simulink model "ADPLL_c7"  (R2017a)
settings: Solver=VariableStepAuto  StartTime=0.0  StopTime=4e-4  FixedStep=1/(12*4*Fref)  RelTol=1e-3
values from neighbouring files (symbols this model uses):
  BBPFD_delay = 1e-09    [processed_29-Aug-2018 09_50_30.mat]    (also in search_0_Kdco-0.9e6_Nref-1e-19_Ndco-1e12.mat; search_0_Kdco-1.0e6_Nref-1e-19_Ndco-1e11.mat; search_0_Kdco-1.0e6_Nref-1e-19_Ndco-1e12.mat; search_0_Kdco-1.0e6_Nref-1e-19_Ndco-1e13.mat)
  DCO_Noise = Datas(i,3)    [CreateDatasetv3.m]    (also in CreateDatasetv4.m; search_0_Kdco-0.9e6_Nref-1e-19_Ndco-1e12.mat = 1000000000000; search_0_Kdco-1.0e6_Nref-1e-19_Ndco-1e11.mat = 100000000000; search_0_Kdco-1.0e6_Nref-1e-19_Ndco-1e12.mat = 1000000000000)
  DCO_Seed = DCO_Seed+1    [CreateDatasetv2.m]    (also in CreateDatasetv3.m = 1; CreateDatasetv4.m = 1; processed_29-Aug-2018 09_50_30.mat = 1; search_0_Kdco-0.9e6_Nref-1e-19_Ndco-1e12.mat = 65)
  Ffree = 255000000    [processed_29-Aug-2018 09_50_30.mat]    (also in search_0_Kdco-0.9e6_Nref-1e-19_Ndco-1e12.mat = 250000000; search_0_Kdco-1.0e6_Nref-1e-19_Ndco-1e11.mat = 250000000; search_0_Kdco-1.0e6_Nref-1e-19_Ndco-1e12.mat = 250000000; search_0_Kdco-1.0e6_Nref-1e-19_Ndco-1e13.mat = 250000000)
  Fref = 25500000    [processed_29-Aug-2018 09_50_30.mat]    (also in search_0_Kdco-0.9e6_Nref-1e-19_Ndco-1e12.mat = 25000000; search_0_Kdco-1.0e6_Nref-1e-19_Ndco-1e11.mat = 25000000; search_0_Kdco-1.0e6_Nref-1e-19_Ndco-1e12.mat = 25000000; search_0_Kdco-1.0e6_Nref-1e-19_Ndco-1e13.mat = 25000000)
  K3 = Datas(i,4)    [CreateDatasetv3.m]    (also in CreateDatasetv4.m)
  K4 = Datas(i,5)    [CreateDatasetv3.m]    (also in CreateDatasetv4.m)
  Kdco = Datas(i,1)    [CreateDatasetv3.m]    (also in CreateDatasetv4.m; search_0_Kdco-0.9e6_Nref-1e-19_Ndco-1e12.mat = 900000; search_0_Kdco-1.0e6_Nref-1e-19_Ndco-1e11.mat = 1000000; search_0_Kdco-1.0e6_Nref-1e-19_Ndco-1e12.mat = 1000000)
  Ki = 0.01    [processed_29-Aug-2018 09_50_30.mat]    (also in search_0_Kdco-0.9e6_Nref-1e-19_Ndco-1e12.mat; search_0_Kdco-1.0e6_Nref-1e-19_Ndco-1e11.mat; search_0_Kdco-1.0e6_Nref-1e-19_Ndco-1e12.mat; search_0_Kdco-1.0e6_Nref-1e-19_Ndco-1e13.mat)
  N = 10    [processed_29-Aug-2018 09_50_30.mat]    (also in search_0_Kdco-0.9e6_Nref-1e-19_Ndco-1e12.mat; search_0_Kdco-1.0e6_Nref-1e-19_Ndco-1e11.mat; search_0_Kdco-1.0e6_Nref-1e-19_Ndco-1e12.mat; search_0_Kdco-1.0e6_Nref-1e-19_Ndco-1e13.mat)
  Ref_Noise = Datas(i,2)    [CreateDatasetv3.m]    (also in CreateDatasetv4.m; search_0_Kdco-0.9e6_Nref-1e-19_Ndco-1e12.mat = 1e-19; search_0_Kdco-1.0e6_Nref-1e-19_Ndco-1e11.mat = 1e-19; search_0_Kdco-1.0e6_Nref-1e-19_Ndco-1e12.mat = 1e-19)
  Ref_Seed = Ref_Seed+1    [CreateDatasetv2.m]    (also in CreateDatasetv3.m = 0; CreateDatasetv4.m = 0; processed_29-Aug-2018 09_50_30.mat = 0; search_0_Kdco-0.9e6_Nref-1e-19_Ndco-1e12.mat = 64)
undefined symbols (not defined in the file): Kp
libraries: simulink_extras x3, dspswit3 x2, simulink x2
settings Model: Creator=ECL328  LastModifiedBy=ECL328

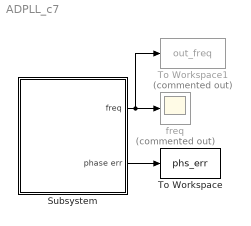
== system ADPLL_c7 ==
  Subsystem : Subsystem  mask{N=N, Kp=Kp, Ki=Ki, Kdco=Kdco, Fref=Fref, Ffree=Ffree, BBPFD_delay=BBPFD_delay, Ref_Noise=Ref_Noise, DCO_Noise=DCO_Noise}
      mask prompts: Ref_Noise "Var of RefNoise"; DCO_Noise "Var of DCONoise"
  To Workspace : ToWorkspace  VariableName=phs_err  SampleTime=-1
  To Workspace1 : ToWorkspace  Commented=on  VariableName=out_freq  SampleTime=-1
  freq : Scope  Commented=on
  wires:
  Subsystem/1(freq) -> To Workspace1/1, freq/1
  Subsystem/2(phase err) -> To Workspace/1

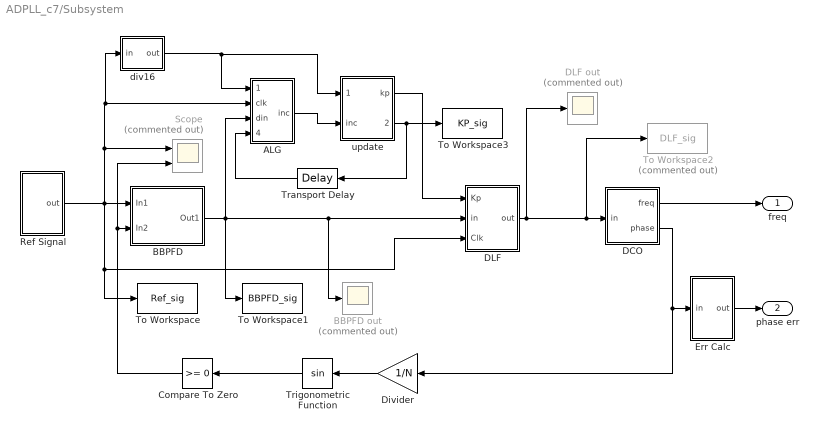
== system ADPLL_c7/Subsystem ==
  ALG : Subsystem
  BBPFD : Subsystem
  BBPFD out : Scope  Commented=on
  Compare To Zero : simulink/Logic and Bit Operations/Compare To Zero  relop=>=  OutDataTypeStr=boolean
  DCO : Subsystem
  DLF : Subsystem
  DLF out : Scope  Commented=on
  Divider : Gain  Gain=1/N
  Err Calc : Subsystem
  Ref Signal : Subsystem
  Scope : Scope  Commented=on  NumInputPorts=2
  To Workspace : ToWorkspace  VariableName=Ref_sig  SampleTime=-1
  To Workspace1 : ToWorkspace  VariableName=BBPFD_sig  SampleTime=-1
  To Workspace2 : ToWorkspace  Commented=on  VariableName=DLF_sig  SampleTime=-1
  To Workspace3 : ToWorkspace  VariableName=KP_sig  SampleTime=-1
  Transport Delay : TransportDelay  DelayTime=BBPFD_delay
  Trigonometric Function : Trigonometry
  div16 : Subsystem
  update : Subsystem
  freq : Outport
  phase err : Outport  Port=2
  wires:
  BBPFD/1(Out1) -> ALG/3(din), To Workspace1/1, DLF/2(in), BBPFD out/1
  Divider/1 -> Trigonometric Function/1
  DLF/1(out) -> DLF out/1, To Workspace2/1, DCO/1(in)
  DCO/1(freq) -> freq/1
  Ref Signal/1(out) -> To Workspace/1, DLF/3(Clk), div16/1(in), ALG/2(clk), Scope/1, BBPFD/1(In1)
  Err Calc/1(out) -> phase err/1
  DCO/2(phase) -> Err Calc/1(in), Divider/1
  Trigonometric Function/1 -> Compare To Zero/1
  Compare To Zero/1 -> Scope/2, BBPFD/2(In2)
  update/1(kp) -> DLF/1(Kp)
  ALG/1(inc) -> update/2(inc)
  update/2(kpraw) -> Transport Delay/1, To Workspace3/1
  Transport Delay/1 -> ALG/4(kpraw)
  div16/1(out) -> update/1("clk16 "), ALG/1(clk16)

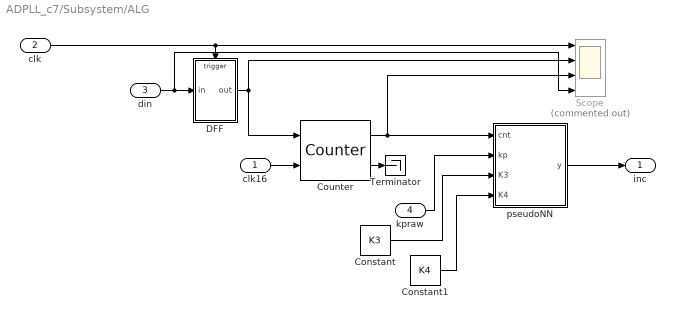
== system ADPLL_c7/Subsystem/ALG ==
  clk16 : Inport
  clk : Inport  Port=2
  din : Inport  Port=3
  kpraw : Inport  Port=4
  Constant : Constant  Value=K3
  Constant1 : Constant  Value=K4
  Counter : dspswit3/Counter  Direction=Up  CountEvent=Rising edge  CounterSize=User defined  MaxCount=1024  InitialCount=0  Output=Count and Hit  HitValue=1024  ResetInput=on  SamplesPerFrame=1  Ts=1  CntDtype=double  HitDtype=Logical
  DFF : Subsystem
  Scope : Scope  Commented=on  NumInputPorts=4
  Terminator : Terminator
  pseudoNN : MATLAB Function  TreatAsAtomicUnit=on
  inc : Outport
  wires:
  Counter/2 -> Terminator/1
  din/1 -> Scope/4, DFF/1(in)
  clk/1 -> Scope/1, DFF/Trigger
  DFF/1(out) -> Scope/2, Counter/1
  Counter/1 -> pseudoNN/1(cnt), Scope/3
  pseudoNN/1(y) -> inc/1
  kpraw/1 -> pseudoNN/2(kp)
  clk16/1 -> Counter/2
  Constant/1 -> pseudoNN/3(K3)
  Constant1/1 -> pseudoNN/4(K4)

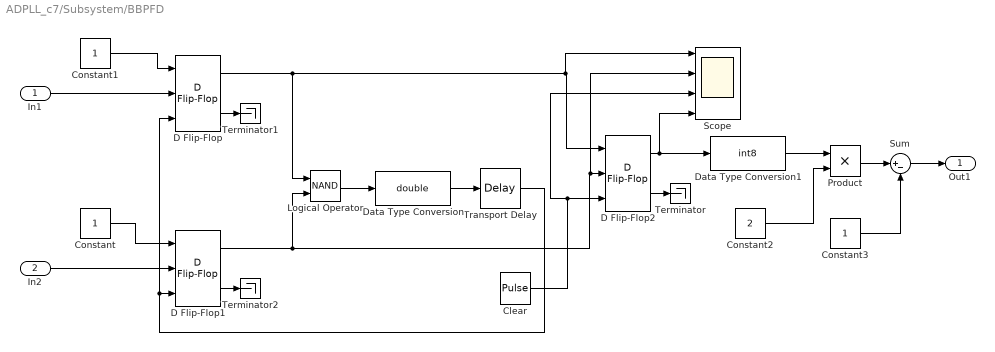
== system ADPLL_c7/Subsystem/BBPFD ==
  In1 : Inport
  In2 : Inport  Port=2
  Clear : DiscretePulseGenerator  PulseType=Time based  Period=20  PulseWidth=50
  Constant : Constant  OutDataTypeStr=boolean
  Constant1 : Constant  OutDataTypeStr=boolean
  Constant2 : Constant  Value=2
  Constant3 : Constant
  D Flip-Flop : simulink_extras/Flip Flops/D Flip-Flop
      settings: SourceProductName=Simulink
  D Flip-Flop1 : simulink_extras/Flip Flops/D Flip-Flop
      settings: SourceProductName=Simulink
  D Flip-Flop2 : simulink_extras/Flip Flops/D Flip-Flop
      settings: SourceProductName=Simulink
  Data Type Conversion : DataTypeConversion  OutDataTypeStr=double
  Data Type Conversion1 : DataTypeConversion  OutDataTypeStr=int8
  Logical Operator : Logic  Operator=NAND  AllPortsSameDT=off  OutDataTypeStr=boolean
  Product : Product
  Scope : Scope  NumInputPorts=4
  Sum : Sum  Inputs=|+-
  Terminator : Terminator
  Terminator1 : Terminator
  Terminator2 : Terminator
  Transport Delay : TransportDelay  DelayTime=BBPFD_delay
  Out1 : Outport
  wires:
  Data Type Conversion/1 -> Transport Delay/1
  Constant/1 -> D Flip-Flop1/1
  Sum/1 -> Out1/1
  D Flip-Flop2/1 -> Scope/4, Data Type Conversion1/1
  Product/1 -> Sum/1
  In1/1 -> D Flip-Flop/2
  Clear/1 -> Scope/3, D Flip-Flop2/3
  D Flip-Flop2/2 -> Terminator/1
  In2/1 -> D Flip-Flop1/2
  Constant3/1 -> Sum/2
  Data Type Conversion1/1 -> Product/1
  Constant1/1 -> D Flip-Flop/1
  Transport Delay/1 -> D Flip-Flop/3, D Flip-Flop1/3
  D Flip-Flop/1 -> Scope/1, D Flip-Flop2/1, Logical Operator/1
  D Flip-Flop1/1 -> Logical Operator/2, Scope/2, D Flip-Flop2/2
  Logical Operator/1 -> Data Type Conversion/1
  D Flip-Flop1/2 -> Terminator2/1
  Constant2/1 -> Product/2
  D Flip-Flop/2 -> Terminator1/1

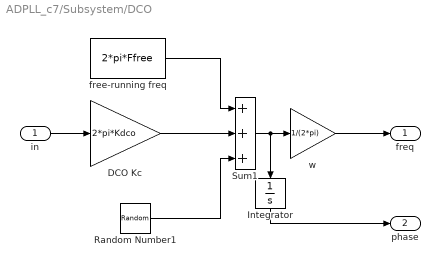
== system ADPLL_c7/Subsystem/DCO ==
  in : Inport
  DCO Kc : Gain  Gain=2*pi*Kdco
  Integrator : Integrator
  Random Number1 : RandomNumber  Variance=DCO_Noise  Seed=DCO_Seed  SampleTime=1/(Fref*4)
  Sum1 : Sum  Inputs=+++
  free-running freq : Constant  Value=2*pi*Ffree
  w : Gain  Gain=1/(2*pi)
  freq : Outport
  phase : Outport  Port=2
  wires:
  in/1 -> DCO Kc/1
  Integrator/1 -> phase/1
  DCO Kc/1 -> Sum1/2
  Sum1/1 -> w/1, Integrator/1
  free-running freq/1 -> Sum1/1
  w/1 -> freq/1
  Random Number1/1 -> Sum1/3

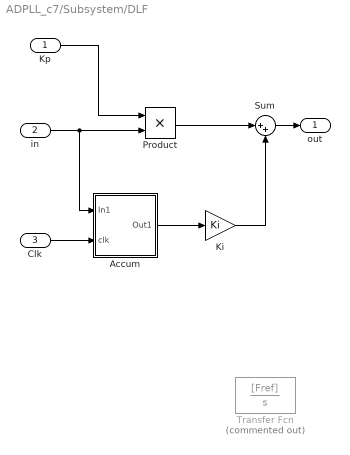
== system ADPLL_c7/Subsystem/DLF ==
  Kp : Inport
  in : Inport  Port=2
  Clk : Inport  Port=3
  Accum : Subsystem
  Ki : Gain  Gain=Ki
  Product : Product
  Sum : Sum  Inputs=|++
  Transfer Fcn : TransferFcn  Commented=on  Numerator=[Fref]  Denominator=[1 0]
  out : Outport
  wires:
  Sum/1 -> out/1
  Clk/1 -> Accum/2(clk)
  Ki/1 -> Sum/2
  Kp/1 -> Product/1
  Accum/1(Out1) -> Ki/1
  in/1 -> Product/2, Accum/1(In1)
  Product/1 -> Sum/1

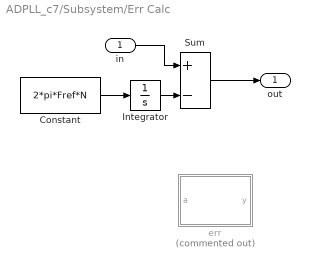
== system ADPLL_c7/Subsystem/Err Calc ==
  in : Inport
  Constant : Constant  Value=2*pi*Fref*N
  Integrator : Integrator
  Sum : Sum  Inputs=+-
  err : MATLAB Function  Commented=on  TreatAsAtomicUnit=on
  out : Outport
  wires:
  Constant/1 -> Integrator/1
  Integrator/1 -> Sum/2
  in/1 -> Sum/1
  Sum/1 -> out/1

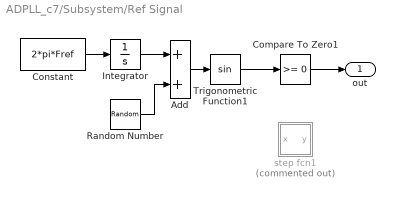
== system ADPLL_c7/Subsystem/Ref Signal ==
  Add : Sum
  Compare To Zero1 : simulink/Logic and Bit Operations/Compare To Zero  relop=>=  OutDataTypeStr=boolean
  Constant : Constant  Value=2*pi*Fref
  Integrator : Integrator
  Random Number : RandomNumber  Variance=Ref_Noise  Seed=Ref_Seed  SampleTime=1/(4*Fref)
  Trigonometric Function1 : Trigonometry
  step fcn1 : Subsystem  Commented=on
  out : Outport
  wires:
  Random Number/1 -> Add/2
  Integrator/1 -> Add/1
  Add/1 -> Trigonometric Function1/1
  Trigonometric Function1/1 -> Compare To Zero1/1
  Compare To Zero1/1 -> out/1
  Constant/1 -> Integrator/1

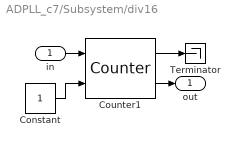
== system ADPLL_c7/Subsystem/div16 ==
  in : Inport
  Constant : Constant
  Counter1 : dspswit3/Counter  Direction=Up  CountEvent=Rising edge  CounterSize=User defined  MaxCount=15  InitialCount=0  Output=Count and Hit  HitValue=15  ResetInput=on  SamplesPerFrame=1  Ts=1  CntDtype=double  HitDtype=Logical
  Terminator : Terminator
  out : Outport
  wires:
  in/1 -> Counter1/1
  Counter1/2 -> out/1
  Constant/1 -> Counter1/2
  Counter1/1 -> Terminator/1

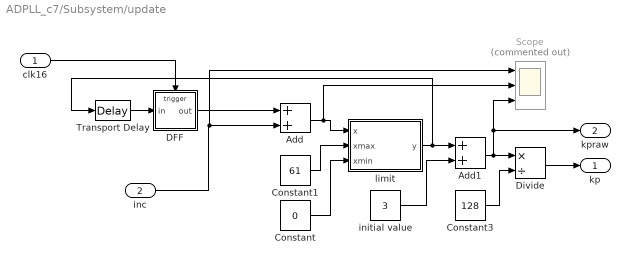
== system ADPLL_c7/Subsystem/update ==
  "clk16 " : Inport
  inc : Inport  Port=2
  Add : Sum
  Add1 : Sum
  Constant : Constant  Value=0
  Constant1 : Constant  Value=61
  Constant3 : Constant  Value=128
  DFF : Subsystem
  Divide : Product  Inputs=*/
  Scope : Scope  Commented=on  NumInputPorts=3
  Transport Delay : TransportDelay  DelayTime=BBPFD_delay
  initial value : Constant  Value=3
  limit : MATLAB Function  TreatAsAtomicUnit=on
  kp : Outport
  kpraw : Outport  Port=2
  wires:
  Divide/1 -> kp/1
  initial value/1 -> Add1/2
  Constant1/1 -> limit/2(xmax)
  Add/1 -> Scope/2, limit/1(x)
  limit/1(y) -> Add1/1, Transport Delay/1
  Constant/1 -> limit/3(xmin)
  inc/1 -> Scope/1, Add/2
  DFF/1(out) -> Add/1
  "clk16 "/1 -> DFF/Trigger
  Transport Delay/1 -> DFF/1(in)
  Add1/1 -> Scope/3, kpraw/1, Divide/1
  Constant3/1 -> Divide/2

== system ADPLL_c7/Subsystem/ALG/DFF ==
  in : Inport
  Trigger : TriggerPort  VariantControl=Variant  PortDimensions=1
  out : Outport
  wires:
  in/1 -> out/1

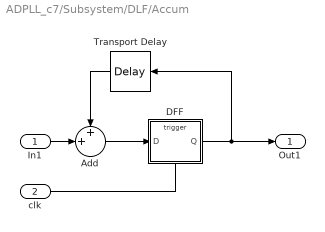
== system ADPLL_c7/Subsystem/DLF/Accum ==
  In1 : Inport
  clk : Inport  Port=2
  Add : Sum  Inputs=++|
  DFF : Subsystem
  Transport Delay : TransportDelay  DelayTime=BBPFD_delay
  Out1 : Outport
  wires:
  In1/1 -> Add/2
  Transport Delay/1 -> Add/1
  Add/1 -> DFF/1(D)
  DFF/1(Q) -> Transport Delay/1, Out1/1
  clk/1 -> DFF/Trigger

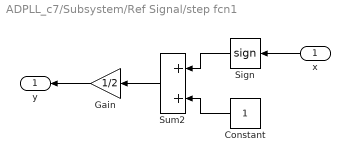
== system ADPLL_c7/Subsystem/Ref Signal/step fcn1 ==
  x : Inport
  Constant : Constant
  Gain : Gain  Gain=1/2
  Sign : Signum
  Sum2 : Sum
  y : Outport
  wires:
  Sum2/1 -> Gain/1
  Gain/1 -> y/1
  x/1 -> Sign/1
  Sign/1 -> Sum2/1
  Constant/1 -> Sum2/2

== system ADPLL_c7/Subsystem/update/DFF ==
  in : Inport
  Trigger : TriggerPort  VariantControl=Variant  PortDimensions=1
  out : Outport
  wires:
  in/1 -> out/1

== system ADPLL_c7/Subsystem/DLF/Accum/DFF ==
  D : Inport
  Trigger : TriggerPort  VariantControl=Variant  PortDimensions=1
  Q : Outport
  wires:
  D/1 -> Q/1

== matlab function ADPLL_c7/Subsystem/update/limit ==
  data: x input; y output; xmax input; xmin input
function y = fcn(x, xmax, xmin)
y = min(max(x,xmin),xmax);

== matlab function ADPLL_c7/Subsystem/Err Calc/err ==
  data: a input; y output
function y = fcn(a)
temp = rem(a,2*pi);
y = temp - (2*pi)*(temp>pi);

== matlab function ADPLL_c7/Subsystem/ALG/pseudoNN ==
  data: cnt input; y output; kp input; K3 input; K4 input
function y = fcn(cnt,kp,K3,K4)
    y = (cnt==3).*((kp<K3)*2-1)+(cnt==4).*((kp<K4)*2-1)+(cnt<3)-(cnt>4);
end
